simulink model "workshop"  (R2018b)
settings: Solver=FixedStepAuto  StartTime=0.0  StopTime=Inf  RelTol=1e-3  EnableMultiTasking=on
libraries: arduinolib x5
settings Model: SimulationMode=external  ExtModeTrigDuration=2  Creator=Admin  LastModifiedBy=Admin
settings OptimizationCC: EnhancedBackFolding=on  PassReuseOutputArgsAs=Individual arguments  MaxStackSize=64  OptimizeBlockOrder=speed  DifferentSizesBufferReuse=on  OptimizationCustomize=off
settings DebuggingCC: ParameterTunabilityLossMsg=error
settings HardwareCC: ProdBitPerPointer=32  ProdBitPerSizeT=32  ProdBitPerPtrDiffT=32  ProdLargestAtomicInteger=Long  ProdLargestAtomicFloat=Double  ProdWordSize=32  ProdHWDeviceType=ARM Compatible->ARM Cortex
settings SFSimCC: MATLABDynamicMemAlloc=off
settings RTWCC: SystemTargetFile=ert.tlc  HardwareBoard=Arduino Due  TemplateMakefile=ert_default_tmf  GenerateReport=on  Toolchain=Arduino ARM  BuildConfiguration=Faster Runs  IncludeHyperlinkInReport=on  LaunchReport=on  GenerateTraceInfo=on  GenerateTraceReport=on  GenerateTraceReportSl=on  GenerateTraceReportSf=on  GenerateTraceReportEml=on
settings CodeAppCC: ForceParamTrailComments=on  IgnoreCustomStorageClasses=off  OperatorAnnotations=on  SimulinkDataObjDesc=on  SFDataObjDesc=on  InsertBlockDesc=on
settings ERTTargetCC: SupportContinuousTime=on  SupportVariableSizeSignals=on  ExtMode=on  ExtModeMexArgs='127.0.0.1' 0 17725

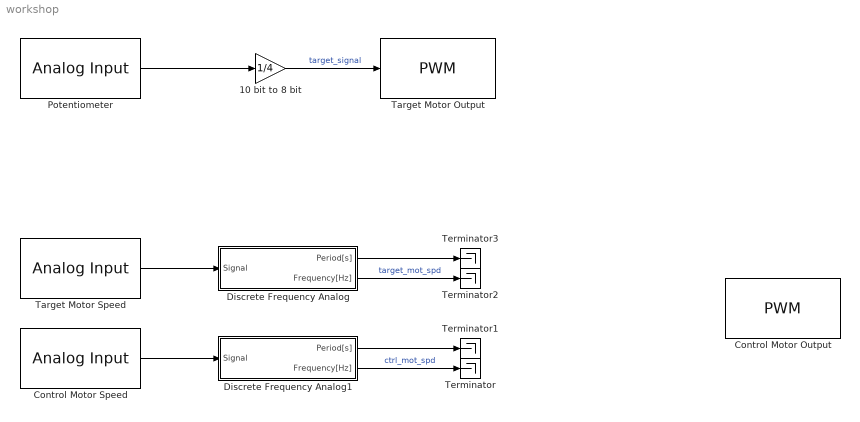
== system workshop ==
  10 bit to 8 bit : Gain  Gain=1/4
  Control Motor Output : arduinolib/PWM  pinNumber=3  EnableInputFrequency=off  InitialFrequency=2000  InitialDutyCycle=0  NotificationType=None  blockPlatform=arduino
  Control Motor Speed : arduinolib/Analog Input  pinNumber=2  ReadResultsOnly=off  ConversionTriggerSource=Software  ExternalTriggerType=uint32(0)  OutputDataType=uint16  EnableConversionCompleteNotify=off  EnableOuputStatus=off  SampleTime=0.001  blockPlatform=arduino
  Discrete Frequency Analog : Subsystem  mask{sampleTime=0.001, threshold=700}
      mask prompts: sampleTime "Sample Time [s]"
  Discrete Frequency Analog1 : Subsystem  mask{sampleTime=0.001, threshold=700}
      mask prompts: sampleTime "Sample Time [s]"
  Potentiometer : arduinolib/Analog Input  pinNumber=0  ReadResultsOnly=off  ConversionTriggerSource=Software  ExternalTriggerType=uint32(0)  OutputDataType=uint16  EnableConversionCompleteNotify=off  EnableOuputStatus=off  SampleTime=0.001  blockPlatform=arduino
  Target Motor Output : arduinolib/PWM  pinNumber=2  EnableInputFrequency=off  InitialFrequency=2000  InitialDutyCycle=0  NotificationType=None  blockPlatform=arduino
  Target Motor Speed : arduinolib/Analog Input  pinNumber=3  ReadResultsOnly=off  ConversionTriggerSource=Software  ExternalTriggerType=uint32(0)  OutputDataType=uint16  EnableConversionCompleteNotify=off  EnableOuputStatus=off  SampleTime=0.001  blockPlatform=arduino
  Terminator{,1..3} (4 alike) : Terminator
  wires:
  Potentiometer/1 -> 10 bit to 8 bit/1
  Target Motor Speed/1 -> Discrete Frequency Analog/1(Signal)
  Control Motor Speed/1 -> Discrete Frequency Analog1/1(Signal)
  10 bit to 8 bit/1 -> Target Motor Output/1  "target_signal"
  Discrete Frequency Analog1/2(Frequency[Hz]) -> Terminator/1  "ctrl_mot_spd"
  Discrete Frequency Analog1/1(Period[s]) -> Terminator1/1
  Discrete Frequency Analog/2(Frequency[Hz]) -> Terminator2/1  "target_mot_spd"
  Discrete Frequency Analog/1(Period[s]) -> Terminator3/1

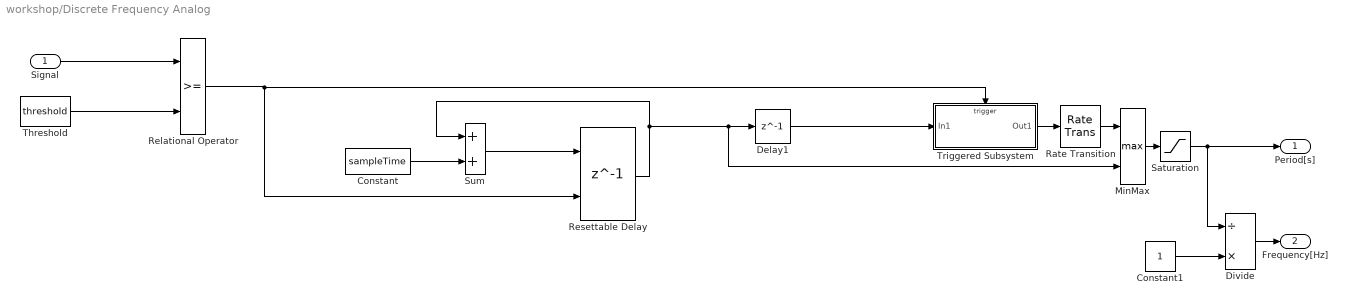
== system workshop/Discrete Frequency Analog ==
  Signal : Inport
  Constant : Constant  Value=sampleTime
  Constant1 : Constant
  Delay1 : Delay  DelayLength=1
  Divide : Product  Inputs=/*
  MinMax : MinMax  Function=max  Inputs=2
  Rate Transition : RateTransition
  Relational Operator : RelationalOperator  OutDataTypeStr=boolean  RndMeth=Simplest
  Resettable Delay : Delay  DelayLength=1  InitialCondition=0  ExternalReset=Rising
      settings: InputPortMap=u0,r5
  Saturation : Saturate  UpperLimit=100  LowerLimit=0.001
  Sum : Sum
  Threshold : Constant  Value=threshold
  Triggered Subsystem : Subsystem  TreatAsAtomicUnit=on
  Period[s] : Outport
  Frequency[Hz] : Outport  Port=2
  wires:
  Divide/1 -> Frequency[Hz]/1
  Constant1/1 -> Divide/2
  Threshold/1 -> Relational Operator/2
  Resettable Delay/1 -> Sum/1, Delay1/1, MinMax/2
  Signal/1 -> Relational Operator/1
  Relational Operator/1 -> Triggered Subsystem/Trigger, Resettable Delay/2
  Sum/1 -> Resettable Delay/1
  Triggered Subsystem/1(Out1) -> Rate Transition/1
  Delay1/1 -> Triggered Subsystem/1(In1)
  Constant/1 -> Sum/2
  Rate Transition/1 -> MinMax/1
  Saturation/1 -> Period[s]/1, Divide/1
  MinMax/1 -> Saturation/1

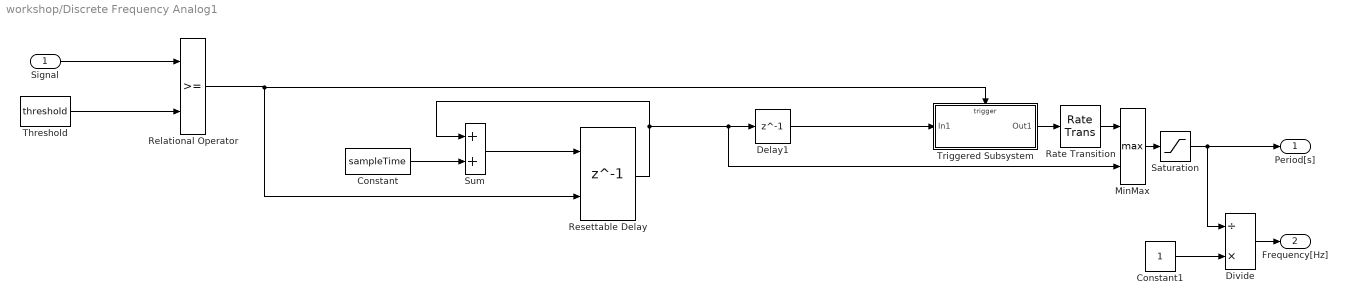
== system workshop/Discrete Frequency Analog1 ==
  Signal : Inport
  Constant : Constant  Value=sampleTime
  Constant1 : Constant
  Delay1 : Delay  DelayLength=1
  Divide : Product  Inputs=/*
  MinMax : MinMax  Function=max  Inputs=2
  Rate Transition : RateTransition
  Relational Operator : RelationalOperator  OutDataTypeStr=boolean  RndMeth=Simplest
  Resettable Delay : Delay  DelayLength=1  InitialCondition=0  ExternalReset=Rising
      settings: InputPortMap=u0,r5
  Saturation : Saturate  UpperLimit=100  LowerLimit=0.001
  Sum : Sum
  Threshold : Constant  Value=threshold
  Triggered Subsystem : Subsystem  TreatAsAtomicUnit=on
  Period[s] : Outport
  Frequency[Hz] : Outport  Port=2
  wires:
  MinMax/1 -> Saturation/1
  Saturation/1 -> Divide/1, Period[s]/1
  Rate Transition/1 -> MinMax/1
  Constant/1 -> Sum/2
  Delay1/1 -> Triggered Subsystem/1(In1)
  Triggered Subsystem/1(Out1) -> Rate Transition/1
  Sum/1 -> Resettable Delay/1
  Relational Operator/1 -> Resettable Delay/2, Triggered Subsystem/Trigger
  Signal/1 -> Relational Operator/1
  Resettable Delay/1 -> MinMax/2, Delay1/1, Sum/1
  Threshold/1 -> Relational Operator/2
  Constant1/1 -> Divide/2
  Divide/1 -> Frequency[Hz]/1

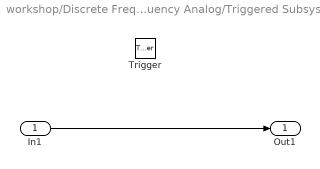
== system workshop/Discrete Frequency Analog/Triggered Subsystem ==
  In1 : Inport
  Trigger : TriggerPort  VariantControl=Variant
  Out1 : Outport
  wires:
  In1/1 -> Out1/1

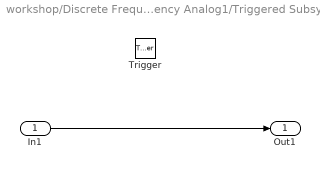
== system workshop/Discrete Frequency Analog1/Triggered Subsystem ==
  In1 : Inport
  Trigger : TriggerPort  VariantControl=Variant
  Out1 : Outport
  wires:
  In1/1 -> Out1/1
